simulink model "c2f_matFile"  (R2019b)
settings: Solver=ode45  StartTime=0.0  StopTime=364  RelTol=1e-3  EnableMultiTasking=on
settings Model: Creator=bbhattac  LastModifiedBy=khung
settings DataIOCC: LimitDataPoints=on  SaveFormat=Array  SignalLoggingSaveFormat=ModelDataLogs  ReturnWorkspaceOutputs=off
settings OptimizationCC: ExpressionDepthLimit=2147483647  LifeSpan=inf
settings DebuggingCC: UnderspecifiedInitializationDetection=Classic  MergeDetectMultiDrivingBlocksExec=none  SolverPrmCheckMsg=warning  FcnCallInpInsideContextMsg=warning  StateNameClashWarn=warning  SFUnexpectedBacktrackingDiag=warning  SFNoUnconditionalDefaultTransitionDiag=warning  SFExecutionAtInitializationDiag=none  ArithmeticOperatorsInVariantConditions=warning
settings HardwareCC: ProdBitPerPointer=32  ProdBitPerSizeT=32  ProdBitPerPtrDiffT=32  ProdLargestAtomicFloat=None  ProdIntDivRoundTo=Undefined  ProdEndianess=Unspecified  ProdWordSize=32  ProdHWDeviceType=32-bit Generic
settings ModelReferenceCC: PropagateSignalLabelsOutOfModel=off
settings SFSimCC: SimUseLocalCustomCode=off
settings RTWCC: RTWUseLocalCustomCode=off
settings CodeAppCC: StateflowObjectComments=on
settings GRTTargetCC: TargetLangStandard=C89/C90 (ANSI)  GeneratePreprocessorConditionals=Disable all  CombineOutputUpdateFcns=off  GRTInterface=on
settings ConfigComp: CovMetricSettings=dw  CovHtmlReporting=on  CovSaveCumulativeToWorkspaceVar=on  CovSaveSingleToWorkspaceVar=on  CovExternalEMLEnable=off

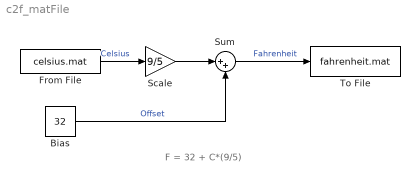
== system c2f_matFile ==
  note: F = 32 + C*(9/5)
  Bias : Constant  Value=32
  From File : FromFile  FileName=celsius.mat  SampleTime=0
  Scale : Gain  Gain=9/5
  Sum : Sum  Inputs=|++
  To File : ToFile  Filename=fahrenheit.mat  MatrixName=outputData
  wires:
  From File/1 -> Scale/1  "Celsius"
  Scale/1 -> Sum/1
  Bias/1 -> Sum/2  "Offset"
  Sum/1 -> To File/1  "Fahrenheit"
